simulink model "rede_SMS"  (Simulink 8.5)
settings: Solver=ode3  StartTime=0.0  StopTime=3  FixedStep=1e-3  MaxStep=1e-3  RelTol=1e-3
libraries: powerlib_extras x4, simulink_need_slupdate x2, AvgModels x1, simulink_extras x1
settings Model: Creator=Batlab  LastModifiedBy=lgalo
settings OptimizationCC: InitFltsAndDblsToZero=on
settings DebuggingCC: SaveWithParameterizedLinksMsg=none  SolverPrmCheckMsg=warning  FcnCallInpInsideContextMsg=UseLocalSettings
settings GRTTargetCC: TargetFcnLib=ansi_tfl_tmw.mat

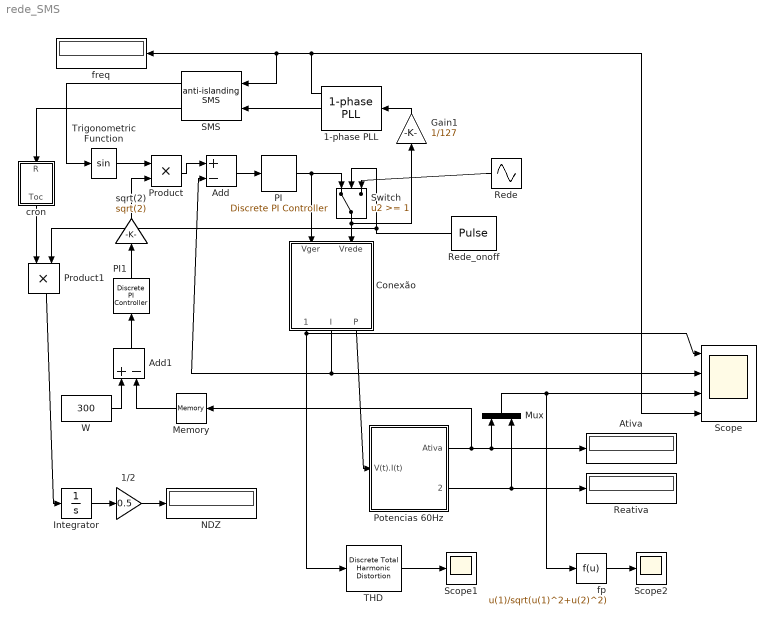
== system rede_SMS ==
  1-phase PLL : powerlib_extras/Control  Blocks/1-phase PLL  Par_Init=[0 60]  ParK=[ 180 3200 1 ]  AGC=off
  1/2 : Gain  Gain=0.5
  Add : Sum  Inputs=+-
  Add1 : Sum  Inputs=+-
  Ativa : Display
  Conexão : Subsystem
  Gain1 : Gain  Gain=1/127
  Integrator : Integrator
  Memory : Memory
  Mux : Mux  Inputs=2
  NDZ : Display
  PI : powerlib_extras/Discrete  Control Blocks/Discrete PI Controller  Kp=10  Ki=20  Par_Limits=[1e3 -1e3]  Init=0  Ts=1e-3
  PI1 : powerlib_extras/Discrete  Control Blocks/Discrete PI Controller  Kp=0.01  Ki=0.05  Par_Limits=[10 0]  Init=0  Ts=1e-3
  Potencias 60Hz : Subsystem
  Product : Product  RndMeth=Zero
  Product1 : Product  RndMeth=Zero
  Reativa : Display
  Rede : Sin  Amplitude=127*sqrt(2)  Frequency=60*2*pi  SampleTime=0
  Rede_onoff : DiscretePulseGenerator  PulseType=Time based  Amplitude=2  PulseWidth=50  PhaseDelay=-1
  SMS : AvgModels/Anti-Ilhamento/anti-islanding SMS  fnom=60  fmax=63  angmax=10
  Scope : Scope  NumInputPorts=4
      settings: TimeRange=3  YMin=-500~-50~-5000~50  YMax=500~50~5000~70  SaveName=dados
  Scope1 : Scope
      settings: TimeRange=3  YMin=-0.3919229176860233  YMax=0.6751100907072167
  Scope2 : Scope
      settings: TimeRange=3  YMin=0.8797282547329597  YMax=1
  Switch : Switch  Threshold=1
  THD : powerlib_extras/Discrete Measurements/Discrete Total Harmonic Distortion  Freq=60  Ts=1e-3
  Trigonometric Function : Trigonometry
  W : Constant  Value=300
  cron : Subsystem
  fp : Fcn  Expr=u(1)/sqrt(u(1)^2+u(2)^2)
  freq : Display
  sqrt(2) : Gain  Gain=sqrt(2)
  wires:
  Conexão/1(Tensões) -> Scope/1, THD/1
  Conexão/3(P) -> Potencias 60Hz/1(V(t).I(t))
  Potencias 60Hz/2(Reativa) -> Reativa/1, Mux/2
  Potencias 60Hz/1(Ativa) -> Ativa/1, Mux/1, Memory/1
  Conexão/2(I) -> Scope/2, Add/2
  Switch/1 -> Conexão/2(Vrede), Gain1/1
  Rede/1 -> Switch/3
  1-phase PLL/1 -> SMS/1, freq/1, Scope/4
  Gain1/1 -> 1-phase PLL/1
  Trigonometric Function/1 -> Product/1
  Rede_onoff/1 -> Switch/2, Product1/2
  Product/1 -> Add/1
  Add/1 -> PI/1
  PI/1 -> Switch/1, Conexão/1(Vger)
  Mux/1 -> Scope/3, fp/1
  SMS/1 -> Trigonometric Function/1
  SMS/2 -> cron/1(R)
  sqrt(2)/1 -> Product/2
  Add1/1 -> PI1/1
  PI1/1 -> sqrt(2)/1
  W/1 -> Add1/1
  Memory/1 -> Add1/2
  Integrator/1 -> 1/2/1
  1/2/1 -> NDZ/1
  Product1/1 -> Integrator/1
  cron/1(Toc) -> Product1/1
  THD/1 -> Scope1/1
  fp/1 -> Scope2/1
  1-phase PLL/2 -> SMS/2

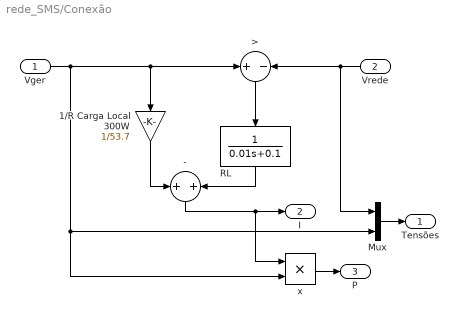
== system rede_SMS/Conexão ==
  Vger : Inport
  Vrede : Inport  Port=2
  - : Sum  Inputs=2
  1/R Carga Local 300W : Gain  Gain=1/53.7
  > : Sum  Inputs=+-
  Mux : Mux  Inputs=2
  RL : TransferFcn  Denominator=[0.01 0.1]
  x : Product  RndMeth=Zero
  Tensões : Outport
  I : Outport  Port=2
  P : Outport  Port=3
  wires:
  Vrede/1 -> Mux/1, >/2
  >/1 -> RL/1
  Vger/1 -> x/2, Mux/2, 1/R Carga Local 300W/1, >/1
  Mux/1 -> Tensões/1
  x/1 -> P/1
  1/R Carga Local 300W/1 -> -/1
  -/1 -> I/1, x/1
  RL/1 -> -/2

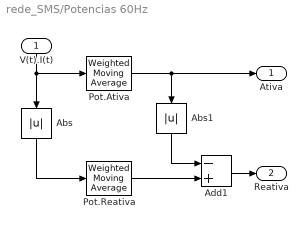
== system rede_SMS/Potencias 60Hz ==
  V(t).I(t) : Inport
  Abs : Abs
  Abs1 : Abs
  Add1 : Sum  Inputs=-+
  Pot.Ativa : simulink_need_slupdate/Weighted Moving Average  mgainval=[ones(1,16)]./16  vinit=0.0  samptime=-1  OutDataType=sfix(16)  OutScaling=2^-10  DoSatur=off  GainDataType=sfix( 16 )  MatRadixGroup=Best Precision: Matrix-wise  GainScaling=2^-10
  Pot.Reativa : simulink_need_slupdate/Weighted Moving Average  mgainval=[ones(1,16)]./16  vinit=0.0  samptime=-1  OutDataType=sfix(16)  OutScaling=2^-10  DoSatur=off  GainDataType=sfix( 16 )  MatRadixGroup=Best Precision: Matrix-wise  GainScaling=2^-10
  Ativa : Outport
  Reativa : Outport  Port=2
  wires:
  Abs/1 -> Pot.Reativa/1
  Pot.Reativa/1 -> Add1/2
  Pot.Ativa/1 -> Abs1/1, Ativa/1
  Abs1/1 -> Add1/1
  V(t).I(t)/1 -> Abs/1, Pot.Ativa/1
  Add1/1 -> Reativa/1

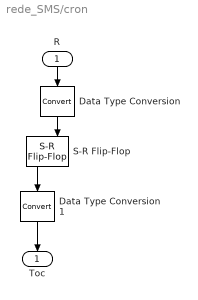
== system rede_SMS/cron ==
  R : Inport
  Data Type Conversion : DataTypeConversion
  Data Type Conversion1 : DataTypeConversion
  S-R Flip-Flop : simulink_extras/Flip Flops/S-R Flip-Flop  initial_condition=1
  Toc : Outport
  wires:
  R/1 -> Data Type Conversion/1
  S-R Flip-Flop/1 -> Data Type Conversion1/1
  Data Type Conversion/1 -> S-R Flip-Flop/2
  Data Type Conversion1/1 -> Toc/1
